simulink model "control_drone"  (R2024b)
settings: Solver=VariableStepAuto  StartTime=0.0  StopTime=10.0  RelTol=1e-3
libraries: simulink x2
settings Model: Creator=schwmaxi  LastModifiedBy=schwmaxi

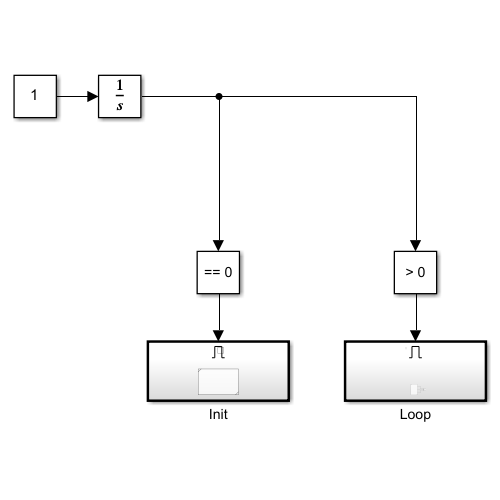
[thumbnail: Simulink's stored preview of the top-level diagram]
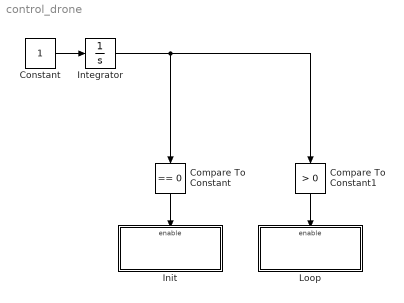
== system control_drone ==
  Compare To Constant : simulink/Logic and Bit Operations/Compare To Constant  relop===  const=0  OutDataTypeStr=boolean
  Compare To Constant1 : simulink/Logic and Bit Operations/Compare To Constant  relop=>  const=0  OutDataTypeStr=boolean
  Constant : Constant
  Init : Subsystem  TreatAsAtomicUnit=on
  Integrator : Integrator
  Loop : Subsystem  TreatAsAtomicUnit=on
  wires:
  Compare To Constant1/1 -> Loop/Enable
  Constant/1 -> Integrator/1
  Integrator/1 -> Compare To Constant1/1, Compare To Constant/1
  Compare To Constant/1 -> Init/Enable

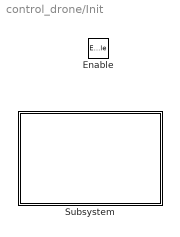
== system control_drone/Init ==
  Enable : EnablePort
  Subsystem : Subsystem  ReferencedSubsystem=InitIMU

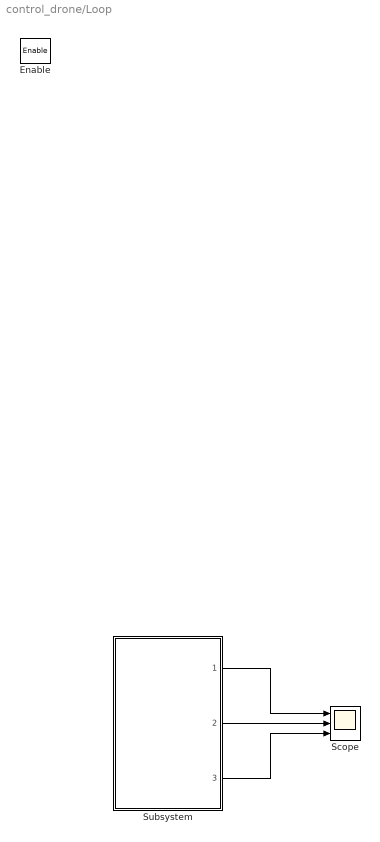
== system control_drone/Loop ==
  Enable : EnablePort
  Scope : Scope  NumInputPorts=3
  Subsystem : Subsystem  ReferencedSubsystem=IMU
  wires:
  Subsystem/2 -> Scope/2
  Subsystem/1 -> Scope/1
  Subsystem/3 -> Scope/3
